simulink model "staubli_20210216_18a"  (R2020a)
settings: Solver=VariableStepAuto  StartTime=0.0  StopTime=10  RelTol=1e-3
values from neighbouring files (symbols this model uses):
  s = T06(1:3,2)    [jacobian_test.m]
undefined symbols (not defined in the file or in its folder): X, Y, Z
libraries: sm_lib x37, nesl_utility x7, dsppolyfun x6, simulink x6
(part 1 of 2)
settings Model: Creator=kdc95  LastModifiedBy=UNIST
settings SolverCC: ZeroCrossAlgorithm=Adaptive
settings DebuggingCC: IgnoredZcDiagnostic=none  ArithmeticOperatorsInVariantConditions=warning
settings SFSimCC: CustomCodeUndefinedFunction=UseInterfaceOnly

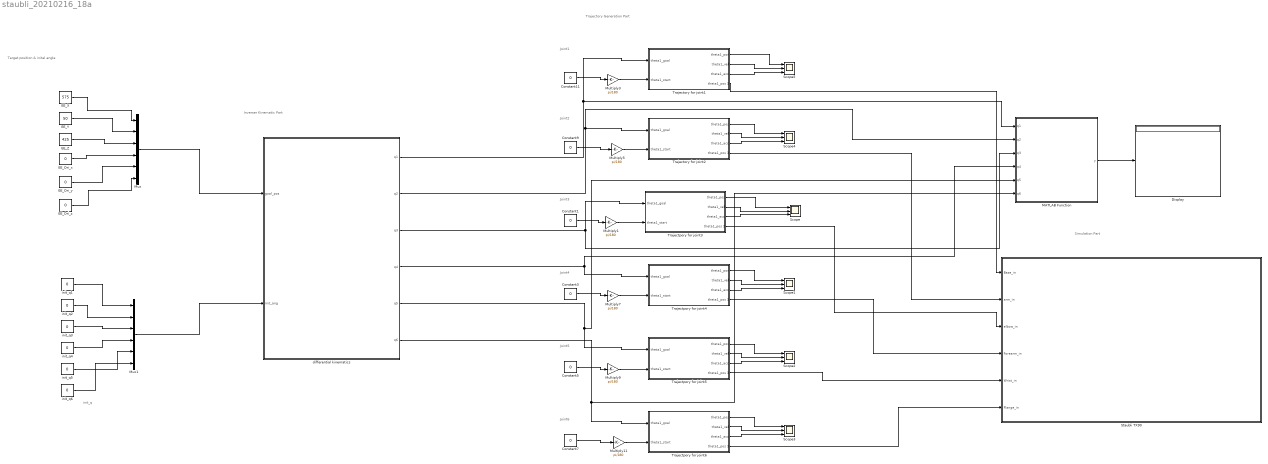
== system staubli_20210216_18a ==
  note: Trajectory Generation Part
  note: init_q
  note: Joint2
  note: Joint3
  note: Joint4
  note: Joint5
  note: Joint1
  note: Joint6
  note: Target position & inital angle
  note: Inverser Kinematic Part
  note: Simulation Part
  Constant{1,3,5,7,9,11} (6 alike) : Constant  Value=0
  Display : Display
  EE_Ori_x : Constant  Value=0
  EE_Ori_y : Constant  Value=0
  EE_Ori_z : Constant  Value=0
  EE_X : Constant  Value=575
  EE_Y : Constant  Value=50
  EE_Z : Constant  Value=425
  MATLAB Function : MATLAB Function  TreatAsAtomicUnit=on
  Multiply{1,3,5,7,9,11} (6 alike) : Gain  Gain=pi/180
  Mux : Mux  Inputs=6
  Mux1 : Mux  Inputs=6
  Scope{,1..5} (6 alike) : Scope  NumInputPorts=3
  Staubli TX90 : Subsystem
      mask Display: image('ROBOT.png'); % Use "Edit Image" on toolstrip to change.
  Trajectory for joint1 : Subsystem
  Trajectory for joint2 : Subsystem
  Trajectpory for joint3 : Subsystem
  Trajectpory for joint4 : Subsystem
  Trajectpory for joint5 : Subsystem
  Trajectpory for joint6 : Subsystem
  differential kinematics : Subsystem
  init_q{1..6} (6 alike) : Constant  Value=0
  wires:
  Trajectpory for joint3/1("theta1_pos ") -> Scope/1
  Trajectory for joint1/3("theta1_acc ") -> Scope5/3
  Trajectpory for joint3/3("theta1_acc ") -> Scope/3
  Constant5/1 -> Multiply9/1
  Trajectpory for joint4/1("theta1_pos ") -> Scope1/1
  Constant11/1 -> Multiply3/1
  Trajectpory for joint5/2("theta1_vel ") -> Scope2/2
  Trajectpory for joint3/2("theta1_vel ") -> Scope/2
  Constant3/1 -> Multiply7/1
  Trajectory for joint1/2("theta1_vel ") -> Scope5/2
  Trajectpory for joint5/1("theta1_pos ") -> Scope2/1
  Trajectpory for joint6/1("theta1_pos ") -> Scope3/1
  Trajectpory for joint5/3("theta1_acc ") -> Scope2/3
  Constant7/1 -> Multiply11/1
  Trajectory for joint2/2("theta1_vel ") -> Scope4/2
  Trajectpory for joint6/3("theta1_acc ") -> Scope3/3
  Trajectory for joint2/1("theta1_pos ") -> Scope4/1
  Trajectory for joint2/3("theta1_acc ") -> Scope4/3
  Trajectpory for joint6/2("theta1_vel ") -> Scope3/2
  Constant1/1 -> Multiply1/1
  Constant9/1 -> Multiply5/1
  Trajectpory for joint4/2("theta1_vel ") -> Scope1/2
  Trajectpory for joint4/3("theta1_acc ") -> Scope1/3
  Trajectory for joint1/1("theta1_pos ") -> Scope5/1
  Trajectory for joint1/4(theta1_pos 1) -> Staubli TX90/1(Base_in)
  Trajectory for joint2/4(theta1_pos 1) -> Staubli TX90/2(arm_in)
  Trajectpory for joint3/4(theta1_pos 1) -> Staubli TX90/3(elbow_in)
  Trajectpory for joint4/4(theta1_pos 1) -> Staubli TX90/4(Forearm_in)
  Trajectpory for joint5/4(theta1_pos 1) -> Staubli TX90/5(Wrist_in)
  Trajectpory for joint6/4(theta1_pos 1) -> Staubli TX90/6(Flange_in)
  differential kinematics/3(q3) -> Trajectpory for joint3/1("theta1_goal "), MATLAB Function/3(q3)
  Multiply1/1 -> Trajectpory for joint3/2("theta1_start ")
  differential kinematics/1(q1) -> Trajectory for joint1/1("theta1_goal "), MATLAB Function/1(q1)
  Multiply3/1 -> Trajectory for joint1/2("theta1_start ")
  differential kinematics/2(q2) -> Trajectory for joint2/1("theta1_goal "), MATLAB Function/2(q2)
  Multiply5/1 -> Trajectory for joint2/2("theta1_start ")
  differential kinematics/4(q4) -> MATLAB Function/4(q4), Trajectpory for joint4/1("theta1_goal ")
  Multiply7/1 -> Trajectpory for joint4/2("theta1_start ")
  differential kinematics/5(q5) -> Trajectpory for joint5/1("theta1_goal "), MATLAB Function/5(q5)
  Multiply9/1 -> Trajectpory for joint5/2("theta1_start ")
  differential kinematics/6(q6) -> Trajectpory for joint6/1("theta1_goal "), MATLAB Function/6(q6)
  Multiply11/1 -> Trajectpory for joint6/2("theta1_start ")
  MATLAB Function/1(y) -> Display/1
  EE_X/1 -> Mux/1
  EE_Y/1 -> Mux/2
  EE_Z/1 -> Mux/3
  EE_Ori_x/1 -> Mux/4
  EE_Ori_y/1 -> Mux/5
  EE_Ori_z/1 -> Mux/6
  init_q1/1 -> Mux1/1
  init_q2/1 -> Mux1/2
  init_q3/1 -> Mux1/3
  init_q4/1 -> Mux1/4
  init_q5/1 -> Mux1/5
  init_q6/1 -> Mux1/6
  Mux/1 -> differential kinematics/1(goal_pos)
  Mux1/1 -> differential kinematics/2(init_ang)

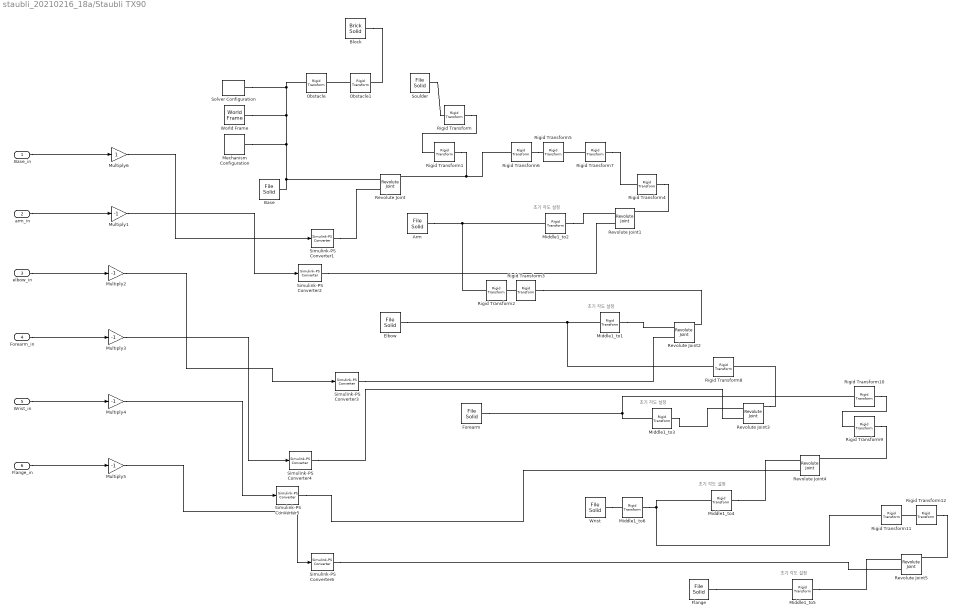
== system staubli_20210216_18a/Staubli TX90 ==
  note: 초기 각도 설정
  note: 초기 각도 설정
  note: 초기 각도 설정
  note: 초기 각도 설정
  note: 초기 각도 설정
  Base_in : Inport
  arm_in : Inport  Port=2
  elbow_in : Inport  Port=3
  Forearm_in : Inport  Port=4
  Wrist_in : Inport  Port=5
  Flange_in : Inport  Port=6
  Arm : sm_lib/Body Elements/File Solid  ExtGeomFileName=C:\Users\UNIST\Desktop\Robot arm\staubli_20210211\arm.stp  UnitType=FromFile  ExtGeomFileUnits=m  StepReaderType=OCC  ExportConvexHullGeometry=off  InertiaType=CalculateFromGeometry  Mass=1  MassUnits=kg  CenterOfMass=[0 0 0]  CenterOfMassUnits=m  MomentsOfInertia=[1 1 1]  MomentsOfInertiaUnits=kg*m^2  ProductsOfInertia=[0 0 0]  ProductsOfInertiaUnits=kg*m^2  BasedOnType=Density  Density=1000  DensityUnits=kg/m^3  DoExposeReferenceFrame=on  SerializedFrames=<Frames/>  GraphicType=FromGeometry  MarkerShape=Sphere  MarkerSize=10  GraphicVisPropType=SimpleVisualProperties  GraphicDiffuseColor=[1.0 1.0 1.0]  GraphicSpecularColor=[0.5 0.5 0.5 1.0]  GraphicAmbientColor=[0.15 0.15 0.15 1.0]  GraphicEmissiveColor=[0.0 0.0 0.0 1.0]  GraphicShininess=75  GraphicOpacity=1
  Base : sm_lib/Body Elements/File Solid  ExtGeomFileName=C:\Users\UNIST\Desktop\Robot arm\staubli_20210211\Base.stp  UnitType=FromFile  ExtGeomFileUnits=m  StepReaderType=HEX  ExportConvexHullGeometry=off  InertiaType=CalculateFromGeometry  Mass=1  MassUnits=kg  CenterOfMass=[0 0 0]  CenterOfMassUnits=m  MomentsOfInertia=[1 1 1]  MomentsOfInertiaUnits=kg*m^2  ProductsOfInertia=[0 0 0]  ProductsOfInertiaUnits=kg*m^2  BasedOnType=Density  Density=1000  DensityUnits=kg/m^3  DoExposeReferenceFrame=on  SerializedFrames=<Frames/>  GraphicType=FromGeometry  MarkerShape=Sphere  MarkerSize=10  GraphicVisPropType=SimpleVisualProperties  GraphicDiffuseColor=[0.5 0.5 0.5]  GraphicSpecularColor=[0.5 0.5 0.5 1.0]  GraphicAmbientColor=[0.15 0.15 0.15 1.0]  GraphicEmissiveColor=[0.0 0.0 0.0 1.0]  GraphicShininess=75  GraphicOpacity=1.0
  Block : sm_lib/Body Elements/Brick Solid  GraphicAmbientColor=[0.15 0.15 0.15 1.0]  BasedOnType=Density  BrickDimensions=[550 400 100]  BrickDimensionUnits=mm  CenterOfMass=[0 0 0]  CenterOfMassUnits=m  GraphicDiffuseColor=[0.5 0.5 0.5]  Density=1000  DensityUnits=kg/m^3  DoExposeReferenceFrame=on  GraphicEmissiveColor=[0.0 0.0 0.0 1.0]  ExportEntireGeometry=off  SerializedFrames=<Frames/>  MarkerShape=Sphere  MarkerSize=10  GraphicType=FromGeometry  InertiaType=CalculateFromGeometry  Mass=1  MassUnits=kg  MomentsOfInertia=[1 1 1]  MomentsOfInertiaUnits=kg*m^2  GraphicOpacity=1.0  ProductsOfInertia=[0 0 0]  ProductsOfInertiaUnits=kg*m^2  GraphicShininess=75  GraphicSpecularColor=[0.5 0.5 0.5 1.0]  GraphicVisPropType=SimpleVisualProperties
  Elbow : sm_lib/Body Elements/File Solid  ExtGeomFileName=C:\Users\UNIST\Desktop\Robot arm\staubli_20210211\Elbow.stp  UnitType=FromFile  ExtGeomFileUnits=m  StepReaderType=OCC  ExportConvexHullGeometry=off  InertiaType=CalculateFromGeometry  Mass=1  MassUnits=kg  CenterOfMass=[0 0 0]  CenterOfMassUnits=m  MomentsOfInertia=[1 1 1]  MomentsOfInertiaUnits=kg*m^2  ProductsOfInertia=[0 0 0]  ProductsOfInertiaUnits=kg*m^2  BasedOnType=Density  Density=1000  DensityUnits=kg/m^3  DoExposeReferenceFrame=on  SerializedFrames=<Frames/>  GraphicType=FromGeometry  MarkerShape=Sphere  MarkerSize=10  GraphicVisPropType=SimpleVisualProperties  GraphicDiffuseColor=[1.0 1.0 1.0]  GraphicSpecularColor=[0.5 0.5 0.5 1.0]  GraphicAmbientColor=[0.15 0.15 0.15 1.0]  GraphicEmissiveColor=[0.0 0.0 0.0 1.0]  GraphicShininess=75  GraphicOpacity=1
  Flange : sm_lib/Body Elements/File Solid  ExtGeomFileName=C:\Users\UNIST\Desktop\Robot arm\staubli_20210211\Flange.stp  UnitType=FromFile  ExtGeomFileUnits=m  StepReaderType=OCC  ExportConvexHullGeometry=off  InertiaType=CalculateFromGeometry  Mass=1  MassUnits=kg  CenterOfMass=[0 0 0]  CenterOfMassUnits=m  MomentsOfInertia=[1 1 1]  MomentsOfInertiaUnits=kg*m^2  ProductsOfInertia=[0 0 0]  ProductsOfInertiaUnits=kg*m^2  BasedOnType=Density  Density=1000  DensityUnits=kg/m^3  DoExposeReferenceFrame=on  SerializedFrames=<Frames/>  GraphicType=FromGeometry  MarkerShape=Sphere  MarkerSize=10  GraphicVisPropType=SimpleVisualProperties  GraphicDiffuseColor=[1.0 1.0 1.0]  GraphicSpecularColor=[0.5 0.5 0.5 1.0]  GraphicAmbientColor=[0.15 0.15 0.15 1.0]  GraphicEmissiveColor=[0.0 0.0 0.0 1.0]  GraphicShininess=75  GraphicOpacity=1
  Forearm : sm_lib/Body Elements/File Solid  ExtGeomFileName=C:\Users\UNIST\Desktop\Robot arm\staubli_20210211\Forearm.stp  UnitType=FromFile  ExtGeomFileUnits=m  StepReaderType=OCC  ExportConvexHullGeometry=off  InertiaType=CalculateFromGeometry  Mass=1  MassUnits=kg  CenterOfMass=[0 0 0]  CenterOfMassUnits=m  MomentsOfInertia=[1 1 1]  MomentsOfInertiaUnits=kg*m^2  ProductsOfInertia=[0 0 0]  ProductsOfInertiaUnits=kg*m^2  BasedOnType=Density  Density=1000  DensityUnits=kg/m^3  DoExposeReferenceFrame=on  SerializedFrames=<Frames/>  GraphicType=FromGeometry  MarkerShape=Sphere  MarkerSize=10  GraphicVisPropType=SimpleVisualProperties  GraphicDiffuseColor=[1.0 1.0 1.0]  GraphicSpecularColor=[0.5 0.5 0.5 1.0]  GraphicAmbientColor=[0.15 0.15 0.15 1.0]  GraphicEmissiveColor=[0.0 0.0 0.0 1.0]  GraphicShininess=75  GraphicOpacity=1
  Mechanism Configuration : sm_lib/Utilities/Mechanism Configuration  UniformGravity=Constant  GravityVector=[0 0 -9.80665]  GravityUnits=m/s^2  LinearizationDelta=0.001
  Middle1_to1 : sm_lib/Frames and Transforms/Rigid Transform  TranslationMethod=None  TranslationStandardOffset=45  TranslationLengthUnit=mm  TranslationStandardAxis=+Z  TranslationCartesianOffset=[0 0 0]  TranslationROffset=0  TranslationROffsetUnits=m  TranslationZOffset=0  TranslationZOffsetUnits=m  TranslationThetaOffset=0  TranslationThetaOffsetUnits=deg  RotationMethod=StandardAxis  RotationAngleUnits=deg  RotationStandardAxis=-Z  RotationAngle=0  RotationArbitraryAxis=[0 0 1]  FollAlignAxisA=+X  BaseAlignAxisA=+Y  FollAlignAxisB=+Y  BaseAlignAxisB=+Z  RotationSequenceAxes=FollowerAxes  RotationSequence=XYX  RotationSequenceAngles=[0 0 0]  RotationSequenceAnglesUnits=deg  RotationMatrix=[1 0 0; 0 1 0; 0 0 1]
  Middle1_to2 : sm_lib/Frames and Transforms/Rigid Transform  TranslationMethod=None  TranslationStandardOffset=45  TranslationLengthUnit=mm  TranslationStandardAxis=+Z  TranslationCartesianOffset=[0 0 0]  TranslationROffset=0  TranslationROffsetUnits=m  TranslationZOffset=0  TranslationZOffsetUnits=m  TranslationThetaOffset=0  TranslationThetaOffsetUnits=deg  RotationMethod=None  RotationAngleUnits=deg  RotationStandardAxis=+Z  RotationAngle=0  RotationArbitraryAxis=[0 0 1]  FollAlignAxisA=+X  BaseAlignAxisA=+Y  FollAlignAxisB=+Y  BaseAlignAxisB=+Z  RotationSequenceAxes=FollowerAxes  RotationSequence=XYX  RotationSequenceAngles=[0 0 0]  RotationSequenceAnglesUnits=deg  RotationMatrix=[1 0 0; 0 1 0; 0 0 1]
  Middle1_to3 : sm_lib/Frames and Transforms/Rigid Transform  TranslationMethod=None  TranslationStandardOffset=45  TranslationLengthUnit=mm  TranslationStandardAxis=+Z  TranslationCartesianOffset=[0 0 0]  TranslationROffset=0  TranslationROffsetUnits=m  TranslationZOffset=0  TranslationZOffsetUnits=m  TranslationThetaOffset=0  TranslationThetaOffsetUnits=deg  RotationMethod=None  RotationAngleUnits=deg  RotationStandardAxis=+Z  RotationAngle=-90  RotationArbitraryAxis=[0 0 1]  FollAlignAxisA=+X  BaseAlignAxisA=+Y  FollAlignAxisB=+Y  BaseAlignAxisB=+Z  RotationSequenceAxes=FollowerAxes  RotationSequence=XYX  RotationSequenceAngles=[0 0 0]  RotationSequenceAnglesUnits=deg  RotationMatrix=[1 0 0; 0 1 0; 0 0 1]
  Middle1_to4 : sm_lib/Frames and Transforms/Rigid Transform  TranslationMethod=None  TranslationStandardOffset=45  TranslationLengthUnit=mm  TranslationStandardAxis=+Z  TranslationCartesianOffset=[0 0 0]  TranslationROffset=0  TranslationROffsetUnits=m  TranslationZOffset=0  TranslationZOffsetUnits=m  TranslationThetaOffset=0  TranslationThetaOffsetUnits=deg  RotationMethod=None  RotationAngleUnits=deg  RotationStandardAxis=-Z  RotationAngle=-90  RotationArbitraryAxis=[0 0 1]  FollAlignAxisA=+X  BaseAlignAxisA=+Y  FollAlignAxisB=+Y  BaseAlignAxisB=+Z  RotationSequenceAxes=FollowerAxes  RotationSequence=XYX  RotationSequenceAngles=[0 0 0]  RotationSequenceAnglesUnits=deg  RotationMatrix=[1 0 0; 0 1 0; 0 0 1]
  Middle1_to5 : sm_lib/Frames and Transforms/Rigid Transform  TranslationMethod=None  TranslationStandardOffset=45  TranslationLengthUnit=mm  TranslationStandardAxis=+Z  TranslationCartesianOffset=[0 0 0]  TranslationROffset=0  TranslationROffsetUnits=m  TranslationZOffset=0  TranslationZOffsetUnits=m  TranslationThetaOffset=0  TranslationThetaOffsetUnits=deg  RotationMethod=None  RotationAngleUnits=deg  RotationStandardAxis=+Z  RotationAngle=-90  RotationArbitraryAxis=[0 0 1]  FollAlignAxisA=+X  BaseAlignAxisA=+Y  FollAlignAxisB=+Y  BaseAlignAxisB=+Z  RotationSequenceAxes=FollowerAxes  RotationSequence=XYX  RotationSequenceAngles=[0 0 0]  RotationSequenceAnglesUnits=deg  RotationMatrix=[1 0 0; 0 1 0; 0 0 1]
  Middle1_to6 : sm_lib/Frames and Transforms/Rigid Transform  TranslationMethod=None  TranslationStandardOffset=45  TranslationLengthUnit=mm  TranslationStandardAxis=+Z  TranslationCartesianOffset=[0 0 0]  TranslationROffset=0  TranslationROffsetUnits=m  TranslationZOffset=0  TranslationZOffsetUnits=m  TranslationThetaOffset=0  TranslationThetaOffsetUnits=deg  RotationMethod=StandardAxis  RotationAngleUnits=deg  RotationStandardAxis=+Z  RotationAngle=-90  RotationArbitraryAxis=[0 0 1]  FollAlignAxisA=+X  BaseAlignAxisA=+Y  FollAlignAxisB=+Y  BaseAlignAxisB=+Z  RotationSequenceAxes=FollowerAxes  RotationSequence=XYX  RotationSequenceAngles=[0 0 0]  RotationSequenceAnglesUnits=deg  RotationMatrix=[1 0 0; 0 1 0; 0 0 1]
  Multiply{1..5} (5 alike) : Gain  Gain=-1
  Multiply6 : Gain
  Obstacle : sm_lib/Frames and Transforms/Rigid Transform  TranslationMethod=StandardAxis  TranslationStandardOffset=700  TranslationLengthUnit=mm  TranslationStandardAxis=+X  TranslationCartesianOffset=[0 0 0]  TranslationROffset=0  TranslationROffsetUnits=m  TranslationZOffset=0  TranslationZOffsetUnits=m  TranslationThetaOffset=0  TranslationThetaOffsetUnits=deg  RotationMethod=None  RotationAngleUnits=deg  RotationStandardAxis=-X  RotationAngle=90  RotationArbitraryAxis=[0 0 1]  FollAlignAxisA=+X  BaseAlignAxisA=+Y  FollAlignAxisB=+Y  BaseAlignAxisB=+Z  RotationSequenceAxes=FollowerAxes  RotationSequence=XYX  RotationSequenceAngles=[0 0 0]  RotationSequenceAnglesUnits=deg  RotationMatrix=[1 0 0; 0 1 0; 0 0 1]
  Obstacle1 : sm_lib/Frames and Transforms/Rigid Transform  TranslationMethod=StandardAxis  TranslationStandardOffset=50  TranslationLengthUnit=mm  TranslationStandardAxis=+Z  TranslationCartesianOffset=[0 0 0]  TranslationROffset=0  TranslationROffsetUnits=m  TranslationZOffset=0  TranslationZOffsetUnits=m  TranslationThetaOffset=0  TranslationThetaOffsetUnits=deg  RotationMethod=None  RotationAngleUnits=deg  RotationStandardAxis=-X  RotationAngle=90  RotationArbitraryAxis=[0 0 1]  FollAlignAxisA=+X  BaseAlignAxisA=+Y  FollAlignAxisB=+Y  BaseAlignAxisB=+Z  RotationSequenceAxes=FollowerAxes  RotationSequence=XYX  RotationSequenceAngles=[0 0 0]  RotationSequenceAnglesUnits=deg  RotationMatrix=[1 0 0; 0 1 0; 0 0 1]
  Revolute Joint{,1..5} (6 alike) : sm_lib/Joints/Revolute Joint  JointMode=Normal  SenseConstraintForce=off  SenseConstraintForceX=off  SenseConstraintForceY=off  SenseConstraintForceZ=off  SenseConstraintTorque=off  SenseConstraintTorqueX=off  SenseConstraintTorqueY=off  SenseConstraintTorqueZ=off  SenseTotalForce=off  SenseTotalForceX=off  SenseTotalForceY=off  SenseTotalForceZ=off  SenseTotalTorque=off  SenseTotalTorqueX=off  SenseTotalTorqueY=off  SenseTotalTorqueZ=off  CompositeWrenchDir=FollowerOnBase  CompositeWrenchFrame=BaseFrame  EquilibriumPosition=0  EquilibriumPositionUnits=deg  SpringStiffness=0  SpringStiffnessUnits=N*m/deg  DampingCoefficient=0.1  DampingCoefficientUnits=N*m/(deg/s)  TorqueActuationMode=ComputedTorque  MotionActuationMode=InputMotion  SensePosition=on  SenseVelocity=off  SenseAcceleration=off  SenseTorqueForce=on  SenseLowerLimitTorqueForce=off  SenseUpperLimitTorqueForce=off  LowerLimitSpecify=off  LowerLimitBound=-90  LowerLimitBoundUnits=deg  LowerLimitStiffness=1e4  LowerLimitStiffnessUnits=N*m/deg  LowerLimitDamping=10  LowerLimitDampingUnits=N*m/(deg/s)  LowerLimitTransitionRegionWidth=0.1  LowerLimitTransitionRegionWidthUnits=deg  UpperLimitSpecify=off  UpperLimitBound=90  UpperLimitBoundUnits=deg  UpperLimitStiffness=1e4  UpperLimitStiffnessUnits=N*m/deg  UpperLimitDamping=10  UpperLimitDampingUnits=N*m/(deg/s)  UpperLimitTransitionRegionWidth=0.1  UpperLimitTransitionRegionWidthUnits=deg  PositionTargetSpecify=off  PositionTargetPriority=High  PositionTargetValue=0  PositionTargetValueUnits=deg  VelocityTargetSpecify=off  VelocityTargetPriority=High  VelocityTargetValue=0  VelocityTargetValueUnits=deg/s
  Rigid Transform : sm_lib/Frames and Transforms/Rigid Transform  TranslationMethod=StandardAxis  TranslationStandardOffset=478  TranslationLengthUnit=mm  TranslationStandardAxis=-Z  TranslationCartesianOffset=[0 0 0]  TranslationROffset=0  TranslationROffsetUnits=m  TranslationZOffset=0  TranslationZOffsetUnits=m  TranslationThetaOffset=0  TranslationThetaOffsetUnits=deg  RotationMethod=None  RotationAngleUnits=deg  RotationStandardAxis=+Z  RotationAngle=0.0  RotationArbitraryAxis=[0 0 1]  FollAlignAxisA=+X  BaseAlignAxisA=+Y  FollAlignAxisB=+Y  BaseAlignAxisB=+Z  RotationSequenceAxes=FollowerAxes  RotationSequence=XYX  RotationSequenceAngles=[0 0 0]  RotationSequenceAnglesUnits=deg  RotationMatrix=[1 0 0; 0 1 0; 0 0 1]
  Rigid Transform1 : sm_lib/Frames and Transforms/Rigid Transform  TranslationMethod=None  TranslationStandardOffset=50  TranslationLengthUnit=mm  TranslationStandardAxis=-X  TranslationCartesianOffset=[0 0 0]  TranslationROffset=0  TranslationROffsetUnits=m  TranslationZOffset=0  TranslationZOffsetUnits=m  TranslationThetaOffset=0  TranslationThetaOffsetUnits=deg  RotationMethod=None  RotationAngleUnits=deg  RotationStandardAxis=+Z  RotationAngle=0.0  RotationArbitraryAxis=[0 0 1]  FollAlignAxisA=+X  BaseAlignAxisA=+Y  FollAlignAxisB=+Y  BaseAlignAxisB=+Z  RotationSequenceAxes=FollowerAxes  RotationSequence=XYX  RotationSequenceAngles=[0 0 0]  RotationSequenceAnglesUnits=deg  RotationMatrix=[1 0 0; 0 1 0; 0 0 1]
  Rigid Transform10 : sm_lib/Frames and Transforms/Rigid Transform  TranslationMethod=None  TranslationStandardOffset=425  TranslationLengthUnit=mm  TranslationStandardAxis=-Y  TranslationCartesianOffset=[0 0 0]  TranslationROffset=0  TranslationROffsetUnits=m  TranslationZOffset=0  TranslationZOffsetUnits=m  TranslationThetaOffset=0  TranslationThetaOffsetUnits=deg  RotationMethod=StandardAxis  RotationAngleUnits=deg  RotationStandardAxis=-X  RotationAngle=90  RotationArbitraryAxis=[0 0 1]  FollAlignAxisA=+X  BaseAlignAxisA=+Y  FollAlignAxisB=+Y  BaseAlignAxisB=+Z  RotationSequenceAxes=FollowerAxes  RotationSequence=XYX  RotationSequenceAngles=[0 0 0]  RotationSequenceAnglesUnits=deg  RotationMatrix=[1 0 0; 0 1 0; 0 0 1]
  Rigid Transform11 : sm_lib/Frames and Transforms/Rigid Transform  TranslationMethod=None  TranslationStandardOffset=425  TranslationLengthUnit=mm  TranslationStandardAxis=-Y  TranslationCartesianOffset=[0 0 0]  TranslationROffset=0  TranslationROffsetUnits=m  TranslationZOffset=0  TranslationZOffsetUnits=m  TranslationThetaOffset=0  TranslationThetaOffsetUnits=deg  RotationMethod=StandardAxis  RotationAngleUnits=deg  RotationStandardAxis=+X  RotationAngle=90  RotationArbitraryAxis=[0 0 1]  FollAlignAxisA=+X  BaseAlignAxisA=+Y  FollAlignAxisB=+Y  BaseAlignAxisB=+Z  RotationSequenceAxes=FollowerAxes  RotationSequence=XYX  RotationSequenceAngles=[0 0 0]  RotationSequenceAnglesUnits=deg  RotationMatrix=[1 0 0; 0 1 0; 0 0 1]
  Rigid Transform12 : sm_lib/Frames and Transforms/Rigid Transform  TranslationMethod=StandardAxis  TranslationStandardOffset=100  TranslationLengthUnit=mm  TranslationStandardAxis=+Z  TranslationCartesianOffset=[0 0 0]  TranslationROffset=0  TranslationROffsetUnits=m  TranslationZOffset=0  TranslationZOffsetUnits=m  TranslationThetaOffset=0  TranslationThetaOffsetUnits=deg  RotationMethod=None  RotationAngleUnits=deg  RotationStandardAxis=+Z  RotationAngle=425  RotationArbitraryAxis=[0 0 1]  FollAlignAxisA=+X  BaseAlignAxisA=+Y  FollAlignAxisB=+Y  BaseAlignAxisB=+Z  RotationSequenceAxes=FollowerAxes  RotationSequence=XYX  RotationSequenceAngles=[0 0 0]  RotationSequenceAnglesUnits=deg  RotationMatrix=[1 0 0; 0 1 0; 0 0 1]
  Rigid Transform2 : sm_lib/Frames and Transforms/Rigid Transform  TranslationMethod=StandardAxis  TranslationStandardOffset=425  TranslationLengthUnit=mm  TranslationStandardAxis=-Y  TranslationCartesianOffset=[0 0 0]  TranslationROffset=0  TranslationROffsetUnits=m  TranslationZOffset=0  TranslationZOffsetUnits=m  TranslationThetaOffset=0  TranslationThetaOffsetUnits=deg  RotationMethod=None  RotationAngleUnits=deg  RotationStandardAxis=+X  RotationAngle=90  RotationArbitraryAxis=[0 0 1]  FollAlignAxisA=+X  BaseAlignAxisA=+Y  FollAlignAxisB=+Y  BaseAlignAxisB=+Z  RotationSequenceAxes=FollowerAxes  RotationSequence=XYX  RotationSequenceAngles=[0 0 0]  RotationSequenceAnglesUnits=deg  RotationMatrix=[1 0 0; 0 1 0; 0 0 1]
  Rigid Transform3 : sm_lib/Frames and Transforms/Rigid Transform  TranslationMethod=StandardAxis  TranslationStandardOffset=50  TranslationLengthUnit=mm  TranslationStandardAxis=+Z  TranslationCartesianOffset=[0 0 0]  TranslationROffset=0  TranslationROffsetUnits=m  TranslationZOffset=0  TranslationZOffsetUnits=m  TranslationThetaOffset=0  TranslationThetaOffsetUnits=deg  RotationMethod=None  RotationAngleUnits=deg  RotationStandardAxis=+X  RotationAngle=90  RotationArbitraryAxis=[0 0 1]  FollAlignAxisA=+X  BaseAlignAxisA=+Y  FollAlignAxisB=+Y  BaseAlignAxisB=+Z  RotationSequenceAxes=FollowerAxes  RotationSequence=XYX  RotationSequenceAngles=[0 0 0]  RotationSequenceAnglesUnits=deg  RotationMatrix=[1 0 0; 0 1 0; 0 0 1]
  Rigid Transform4 : sm_lib/Frames and Transforms/Rigid Transform  TranslationMethod=StandardAxis  TranslationStandardOffset=50  TranslationLengthUnit=mm  TranslationStandardAxis=+X  TranslationCartesianOffset=[0 0 0]  TranslationROffset=0  TranslationROffsetUnits=m  TranslationZOffset=0  TranslationZOffsetUnits=m  TranslationThetaOffset=0  TranslationThetaOffsetUnits=deg  RotationMethod=None  RotationAngleUnits=deg  RotationStandardAxis=+X  RotationAngle=90  RotationArbitraryAxis=[0 0 1]  FollAlignAxisA=+X  BaseAlignAxisA=+Y  FollAlignAxisB=+Y  BaseAlignAxisB=+Z  RotationSequenceAxes=FollowerAxes  RotationSequence=XYX  RotationSequenceAngles=[0 0 0]  RotationSequenceAnglesUnits=deg  RotationMatrix=[1 0 0; 0 1 0; 0 0 1]
  Rigid Transform5 : sm_lib/Frames and Transforms/Rigid Transform  TranslationMethod=StandardAxis  TranslationStandardOffset=425  TranslationLengthUnit=mm  TranslationStandardAxis=-Y  TranslationCartesianOffset=[0 0 0]  TranslationROffset=0  TranslationROffsetUnits=m  TranslationZOffset=0  TranslationZOffsetUnits=m  TranslationThetaOffset=0  TranslationThetaOffsetUnits=deg  RotationMethod=None  RotationAngleUnits=deg  RotationStandardAxis=+X  RotationAngle=90  RotationArbitraryAxis=[0 0 1]  FollAlignAxisA=+X  BaseAlignAxisA=+Y  FollAlignAxisB=+Y  BaseAlignAxisB=+Z  RotationSequenceAxes=FollowerAxes  RotationSequence=XYX  RotationSequenceAngles=[0 0 0]  RotationSequenceAnglesUnits=deg  RotationMatrix=[1 0 0; 0 1 0; 0 0 1]
  Rigid Transform6 : sm_lib/Frames and Transforms/Rigid Transform  TranslationMethod=None  TranslationStandardOffset=50  TranslationLengthUnit=mm  TranslationStandardAxis=-X  TranslationCartesianOffset=[0 0 0]  TranslationROffset=0  TranslationROffsetUnits=m  TranslationZOffset=0  TranslationZOffsetUnits=m  TranslationThetaOffset=0  TranslationThetaOffsetUnits=deg  RotationMethod=StandardAxis  RotationAngleUnits=deg  RotationStandardAxis=-X  RotationAngle=90  RotationArbitraryAxis=[0 0 1]  FollAlignAxisA=+X  BaseAlignAxisA=+Y  FollAlignAxisB=+Y  BaseAlignAxisB=+Z  RotationSequenceAxes=FollowerAxes  RotationSequence=XYX  RotationSequenceAngles=[0 0 0]  RotationSequenceAnglesUnits=deg  RotationMatrix=[1 0 0; 0 1 0; 0 0 1]
  Rigid Transform7 : sm_lib/Frames and Transforms/Rigid Transform  TranslationMethod=StandardAxis  TranslationStandardOffset=50  TranslationLengthUnit=mm  TranslationStandardAxis=-Y  TranslationCartesianOffset=[0 0 0]  TranslationROffset=0  TranslationROffsetUnits=m  TranslationZOffset=0  TranslationZOffsetUnits=m  TranslationThetaOffset=0  TranslationThetaOffsetUnits=deg  RotationMethod=None  RotationAngleUnits=deg  RotationStandardAxis=+X  RotationAngle=90  RotationArbitraryAxis=[0 0 1]  FollAlignAxisA=+X  BaseAlignAxisA=+Y  FollAlignAxisB=+Y  BaseAlignAxisB=+Z  RotationSequenceAxes=FollowerAxes  RotationSequence=XYX  RotationSequenceAngles=[0 0 0]  RotationSequenceAnglesUnits=deg  RotationMatrix=[1 0 0; 0 1 0; 0 0 1]
  Rigid Transform8 : sm_lib/Frames and Transforms/Rigid Transform  TranslationMethod=None  TranslationStandardOffset=425  TranslationLengthUnit=mm  TranslationStandardAxis=-Y  TranslationCartesianOffset=[0 0 0]  TranslationROffset=0  TranslationROffsetUnits=m  TranslationZOffset=0  TranslationZOffsetUnits=m  TranslationThetaOffset=0  TranslationThetaOffsetUnits=deg  RotationMethod=StandardAxis  RotationAngleUnits=deg  RotationStandardAxis=+X  RotationAngle=90  RotationArbitraryAxis=[0 0 1]  FollAlignAxisA=+X  BaseAlignAxisA=+Y  FollAlignAxisB=+Y  BaseAlignAxisB=+Z  RotationSequenceAxes=FollowerAxes  RotationSequence=XYX  RotationSequenceAngles=[0 0 0]  RotationSequenceAnglesUnits=deg  RotationMatrix=[1 0 0; 0 1 0; 0 0 1]
  Rigid Transform9 : sm_lib/Frames and Transforms/Rigid Transform  TranslationMethod=StandardAxis  TranslationStandardOffset=425  TranslationLengthUnit=mm  TranslationStandardAxis=-Y  TranslationCartesianOffset=[0 0 0]  TranslationROffset=0  TranslationROffsetUnits=m  TranslationZOffset=0  TranslationZOffsetUnits=m  TranslationThetaOffset=0  TranslationThetaOffsetUnits=deg  RotationMethod=None  RotationAngleUnits=deg  RotationStandardAxis=+Z  RotationAngle=425  RotationArbitraryAxis=[0 0 1]  FollAlignAxisA=+X  BaseAlignAxisA=+Y  FollAlignAxisB=+Y  BaseAlignAxisB=+Z  RotationSequenceAxes=FollowerAxes  RotationSequence=XYX  RotationSequenceAngles=[0 0 0]  RotationSequenceAnglesUnits=deg  RotationMatrix=[1 0 0; 0 1 0; 0 0 1]
  Simulink-PS Converter{1..6} (6 alike) : nesl_utility/Simulink-PS Converter  PhysicalDomain=network_engine_domain  SubClassName=ps_input  LeftPortType=input  RightPortType=output  PseudoPeriodic=off  Frequencies=[]  NoiseDistribution=none  NoiseParameters=[]  Unit=1  AffineConversion=off  FilteringAndDerivatives=filter  SimscapeFilterOrder=2  InputFilterTimeConstant=0.1  UdotUserProvided=0
  Solver Configuration : nesl_utility/Solver Configuration  PhysicalDomain=network_engine_domain  SubClassName=solver  LeftPortType=input  RightPortType=generic  Tones=[]  Harmonics=[]  SimulateNoise=off  Profile=off  UseLocalSampling=off  EnableSwitchedLinearOptims=on  FrequencyDomain=off  UseCCode=off  RelTol=0.001  AbsTol=1e-06  MinStep=1e-09  ToWorkspace=off  RevertToSquareIcSolve=off  NumHomotopyIterations=100  PhasorMode=off  PhasorModeNumHarmonics=1  DoDC=off  ResidualTolerance=1e-09  UseLocalSolver=off  LocalSolverChoice=NE_BACKWARD_EULER_ADVANCER  LocalSolverSampleTime=0.001  DoFixedCost=off  MaxNonlinIter=3  MaxModeIter=2  LinearAlgebra=auto  EquationFormulation=NE_TIME_EF  DelaysMemoryBudget=1024  AutomaticFiltering=on  FilteringTimeConstant=0.001  PartitionStorageMethod=AS_NEEDED  PartitionMemoryBudget=1024  PartitionMethod=ROBUST
  Soulder : sm_lib/Body Elements/File Solid  ExtGeomFileName=C:\Users\UNIST\Desktop\Robot arm\staubli_20210211\Shoulder.stp  UnitType=FromFile  ExtGeomFileUnits=m  StepReaderType=HEX  ExportConvexHullGeometry=off  InertiaType=CalculateFromGeometry  Mass=1  MassUnits=kg  CenterOfMass=[0 0 0]  CenterOfMassUnits=m  MomentsOfInertia=[1 1 1]  MomentsOfInertiaUnits=kg*m^2  ProductsOfInertia=[0 0 0]  ProductsOfInertiaUnits=kg*m^2  BasedOnType=Density  Density=1000  DensityUnits=kg/m^3  DoExposeReferenceFrame=on  SerializedFrames=<Frames/>  GraphicType=FromGeometry  MarkerShape=Sphere  MarkerSize=10  GraphicVisPropType=SimpleVisualProperties  GraphicDiffuseColor=[0.5 0.5 0.5]  GraphicSpecularColor=[0.5 0.5 0.5 1.0]  GraphicAmbientColor=[0.15 0.15 0.15 1.0]  GraphicEmissiveColor=[0.0 0.0 0.0 1.0]  GraphicShininess=75  GraphicOpacity=1.0
  World Frame : sm_lib/Frames and Transforms/World Frame
  Wrist : sm_lib/Body Elements/File Solid  ExtGeomFileName=C:\Users\UNIST\Desktop\Robot arm\staubli_20210211\Wrist.stp  UnitType=FromFile  ExtGeomFileUnits=m  StepReaderType=OCC  ExportConvexHullGeometry=off  InertiaType=CalculateFromGeometry  Mass=1  MassUnits=kg  CenterOfMass=[0 0 0]  CenterOfMassUnits=m  MomentsOfInertia=[1 1 1]  MomentsOfInertiaUnits=kg*m^2  ProductsOfInertia=[0 0 0]  ProductsOfInertiaUnits=kg*m^2  BasedOnType=Density  Density=1000  DensityUnits=kg/m^3  DoExposeReferenceFrame=on  SerializedFrames=<Frames/>  GraphicType=FromGeometry  MarkerShape=Sphere  MarkerSize=10  GraphicVisPropType=SimpleVisualProperties  GraphicDiffuseColor=[1.0 1.0 1.0]  GraphicSpecularColor=[0.5 0.5 0.5 1.0]  GraphicAmbientColor=[0.15 0.15 0.15 1.0]  GraphicEmissiveColor=[0.0 0.0 0.0 1.0]  GraphicShininess=75  GraphicOpacity=1
  wires:
  arm_in/1 -> Multiply1/1
  elbow_in/1 -> Multiply2/1
  Wrist_in/1 -> Multiply4/1
  Forearm_in/1 -> Multiply3/1
  Base_in/1 -> Multiply6/1
  Multiply1/1 -> Simulink-PS Converter2/1
  Multiply2/1 -> Simulink-PS Converter3/1
  Multiply3/1 -> Simulink-PS Converter4/1
  Multiply4/1 -> Simulink-PS Converter5/1
  Multiply5/1 -> Simulink-PS Converter6/1
  Flange_in/1 -> Multiply5/1
  Multiply6/1 -> Simulink-PS Converter1/1
  connections:
  Solver Configuration/RConn1 -- Revolute Joint/LConn1 -- Base/RConn1 -- Mechanism Configuration/RConn1 -- World Frame/RConn1 -- Obstacle/LConn1
  Block/RConn1 -- Obstacle1/RConn1
  Obstacle1/LConn1 -- Obstacle/RConn1
  Simulink-PS Converter1/RConn1 -- Revolute Joint/LConn2
  Soulder/RConn1 -- Rigid Transform/LConn1
  Rigid Transform/RConn1 -- Rigid Transform1/LConn1
  Rigid Transform1/RConn1 -- Revolute Joint/RConn1 -- Rigid Transform6/LConn1
  Arm/RConn1 -- Rigid Transform2/LConn1 -- Middle1_to2/LConn1
  Simulink-PS Converter2/RConn1 -- Revolute Joint1/LConn2
  Middle1_to2/RConn1 -- Revolute Joint1/LConn1
  Rigid Transform7/LConn1 -- Rigid Transform5/RConn1
  Rigid Transform6/RConn1 -- Rigid Transform5/LConn1
  Rigid Transform7/RConn1 -- Rigid Transform4/LConn1
  Rigid Transform4/RConn1 -- Revolute Joint1/RConn1
  Elbow/RConn1 -- Rigid Transform8/LConn1 -- Middle1_to1/LConn1
  Rigid Transform3/LConn1 -- Rigid Transform2/RConn1
  Rigid Transform3/RConn1 -- Revolute Joint2/RConn1
  Simulink-PS Converter3/RConn1 -- Revolute Joint2/LConn2
  Middle1_to1/RConn1 -- Revolute Joint2/LConn1
  Forearm/RConn1 -- Middle1_to3/LConn1 -- Rigid Transform10/LConn1
  Middle1_to3/RConn1 -- Revolute Joint3/LConn1
  Revolute Joint3/RConn1 -- Rigid Transform8/RConn1
  Rigid Transform11/LConn1 -- Middle1_to6/RConn1 -- Middle1_to4/LConn1
  Rigid Transform10/RConn1 -- Rigid Transform9/LConn1
  Rigid Transform9/RConn1 -- Revolute Joint4/RConn1
  Middle1_to5/RConn1 -- Revolute Joint5/LConn1
  Flange/RConn1 -- Middle1_to5/LConn1
  Rigid Transform12/LConn1 -- Rigid Transform11/RConn1
  Rigid Transform12/RConn1 -- Revolute Joint5/RConn1
  Simulink-PS Converter4/RConn1 -- Revolute Joint3/LConn2
  Simulink-PS Converter5/RConn1 -- Revolute Joint4/LConn2
  Simulink-PS Converter6/RConn1 -- Revolute Joint5/LConn2
  Middle1_to4/RConn1 -- Revolute Joint4/LConn1
  Wrist/RConn1 -- Middle1_to6/LConn1

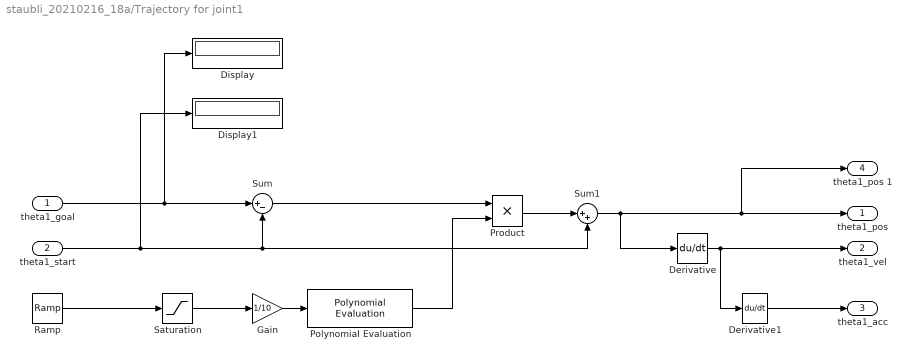
== system staubli_20210216_18a/Trajectory for joint1 ==
  "theta1_goal " : Inport
  "theta1_start " : Inport  Port=2
  Derivative : Derivative
  Derivative1 : Derivative
  Display : Display
  Display1 : Display
  Gain : Gain  Gain=1/10
  Polynomial Evaluation : dsppolyfun/Polynomial Evaluation  useConstCoeffs=on  constCoeffs=[6 -15 10 0 0 0]
      settings: SourceProductBaseCode=DS
  Product : Product
  Ramp : simulink/Sources/Ramp  slope=1  start=0  InitialOutput=0
  Saturation : Saturate  UpperLimit=10  LowerLimit=-10
  Sum : Sum  Inputs=|+-
  Sum1 : Sum  Inputs=|++
  "theta1_pos " : Outport  VectorParamsAs1DForOutWhenUnconnected=off
  "theta1_vel " : Outport  Port=2  VectorParamsAs1DForOutWhenUnconnected=off
  "theta1_acc " : Outport  Port=3  VectorParamsAs1DForOutWhenUnconnected=off
  theta1_pos 1 : Outport  Port=4  VectorParamsAs1DForOutWhenUnconnected=off
  wires:
  "theta1_start "/1 -> Sum1/2, Sum/2, Display1/1
  Sum/1 -> Product/1
  "theta1_goal "/1 -> Display/1, Sum/1
  Sum1/1 -> Derivative/1, theta1_pos 1/1, "theta1_pos "/1
  Derivative/1 -> "theta1_vel "/1, Derivative1/1
  Gain/1 -> Polynomial Evaluation/1
  Product/1 -> Sum1/1
  Polynomial Evaluation/1 -> Product/2
  Derivative1/1 -> "theta1_acc "/1
  Saturation/1 -> Gain/1
  Ramp/1 -> Saturation/1

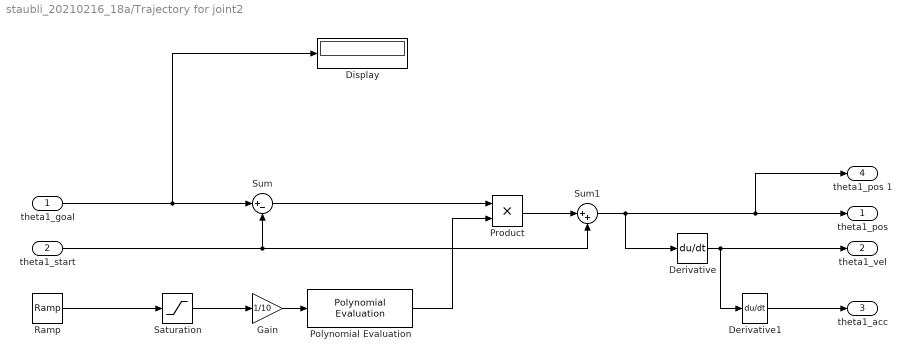
== system staubli_20210216_18a/Trajectory for joint2 ==
  "theta1_goal " : Inport
  "theta1_start " : Inport  Port=2
  Derivative : Derivative
  Derivative1 : Derivative
  Display : Display
  Gain : Gain  Gain=1/10
  Polynomial Evaluation : dsppolyfun/Polynomial Evaluation  useConstCoeffs=on  constCoeffs=[6 -15 10 0 0 0]
      settings: SourceProductBaseCode=DS
  Product : Product
  Ramp : simulink/Sources/Ramp  slope=1  start=0  InitialOutput=0
  Saturation : Saturate  UpperLimit=10  LowerLimit=-10
  Sum : Sum  Inputs=|+-
  Sum1 : Sum  Inputs=|++
  "theta1_pos " : Outport  VectorParamsAs1DForOutWhenUnconnected=off
  "theta1_vel " : Outport  Port=2  VectorParamsAs1DForOutWhenUnconnected=off
  "theta1_acc " : Outport  Port=3  VectorParamsAs1DForOutWhenUnconnected=off
  theta1_pos 1 : Outport  Port=4  VectorParamsAs1DForOutWhenUnconnected=off
  wires:
  "theta1_start "/1 -> Sum1/2, Sum/2
  Sum/1 -> Product/1
  "theta1_goal "/1 -> Display/1, Sum/1
  Sum1/1 -> Derivative/1, theta1_pos 1/1, "theta1_pos "/1
  Derivative/1 -> "theta1_vel "/1, Derivative1/1
  Gain/1 -> Polynomial Evaluation/1
  Product/1 -> Sum1/1
  Polynomial Evaluation/1 -> Product/2
  Derivative1/1 -> "theta1_acc "/1
  Saturation/1 -> Gain/1
  Ramp/1 -> Saturation/1

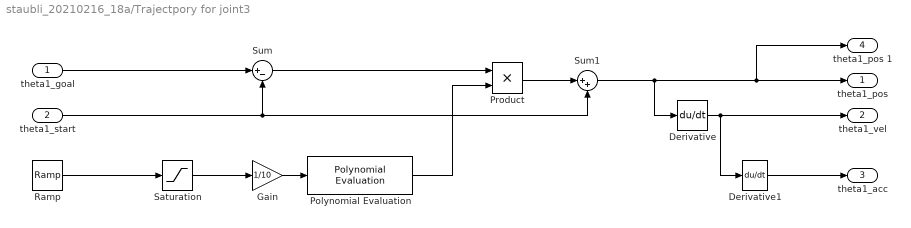
== system staubli_20210216_18a/Trajectpory for joint3 ==
  "theta1_goal " : Inport
  "theta1_start " : Inport  Port=2
  Derivative : Derivative
  Derivative1 : Derivative
  Gain : Gain  Gain=1/10
  Polynomial Evaluation : dsppolyfun/Polynomial Evaluation  useConstCoeffs=on  constCoeffs=[6 -15 10 0 0 0]
      settings: SourceProductBaseCode=DS
  Product : Product
  Ramp : simulink/Sources/Ramp  slope=1  start=0  InitialOutput=0
  Saturation : Saturate  UpperLimit=10  LowerLimit=-10
  Sum : Sum  Inputs=|+-
  Sum1 : Sum  Inputs=|++
  "theta1_pos " : Outport  VectorParamsAs1DForOutWhenUnconnected=off
  "theta1_vel " : Outport  Port=2  VectorParamsAs1DForOutWhenUnconnected=off
  "theta1_acc " : Outport  Port=3  VectorParamsAs1DForOutWhenUnconnected=off
  theta1_pos 1 : Outport  Port=4  VectorParamsAs1DForOutWhenUnconnected=off
  wires:
  Sum/1 -> Product/1
  Derivative/1 -> "theta1_vel "/1, Derivative1/1
  Gain/1 -> Polynomial Evaluation/1
  Product/1 -> Sum1/1
  Polynomial Evaluation/1 -> Product/2
  Derivative1/1 -> "theta1_acc "/1
  Saturation/1 -> Gain/1
  Ramp/1 -> Saturation/1
  "theta1_goal "/1 -> Sum/1
  "theta1_start "/1 -> Sum1/2, Sum/2
  Sum1/1 -> Derivative/1, theta1_pos 1/1, "theta1_pos "/1

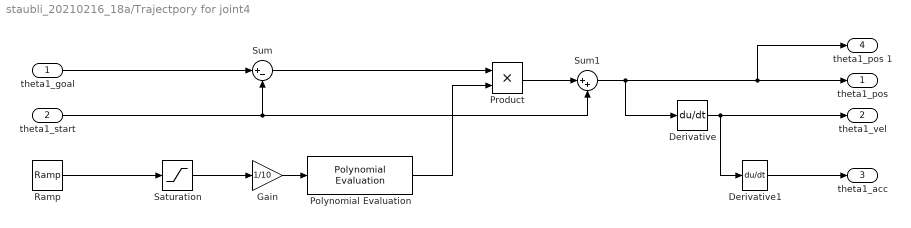
== system staubli_20210216_18a/Trajectpory for joint4 ==
  "theta1_goal " : Inport
  "theta1_start " : Inport  Port=2
  Derivative : Derivative
  Derivative1 : Derivative
  Gain : Gain  Gain=1/10
  Polynomial Evaluation : dsppolyfun/Polynomial Evaluation  useConstCoeffs=on  constCoeffs=[6 -15 10 0 0 0]
      settings: SourceProductBaseCode=DS
  Product : Product
  Ramp : simulink/Sources/Ramp  slope=1  start=0  InitialOutput=0
  Saturation : Saturate  UpperLimit=10  LowerLimit=-10
  Sum : Sum  Inputs=|+-
  Sum1 : Sum  Inputs=|++
  "theta1_pos " : Outport  VectorParamsAs1DForOutWhenUnconnected=off
  "theta1_vel " : Outport  Port=2  VectorParamsAs1DForOutWhenUnconnected=off
  "theta1_acc " : Outport  Port=3  VectorParamsAs1DForOutWhenUnconnected=off
  theta1_pos 1 : Outport  Port=4  VectorParamsAs1DForOutWhenUnconnected=off
  wires:
  "theta1_start "/1 -> Sum1/2, Sum/2
  Sum/1 -> Product/1
  "theta1_goal "/1 -> Sum/1
  Sum1/1 -> Derivative/1, theta1_pos 1/1, "theta1_pos "/1
  Derivative/1 -> "theta1_vel "/1, Derivative1/1
  Gain/1 -> Polynomial Evaluation/1
  Product/1 -> Sum1/1
  Polynomial Evaluation/1 -> Product/2
  Derivative1/1 -> "theta1_acc "/1
  Saturation/1 -> Gain/1
  Ramp/1 -> Saturation/1

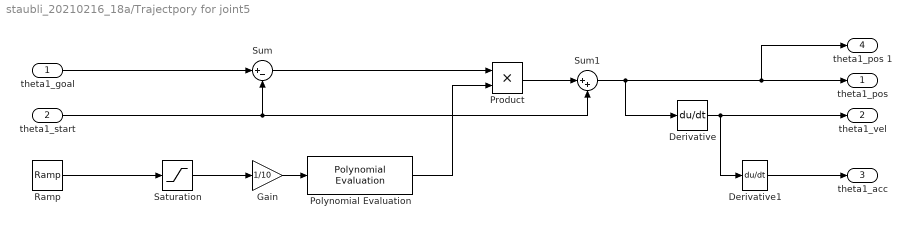
== system staubli_20210216_18a/Trajectpory for joint5 ==
  "theta1_goal " : Inport
  "theta1_start " : Inport  Port=2
  Derivative : Derivative
  Derivative1 : Derivative
  Gain : Gain  Gain=1/10
  Polynomial Evaluation : dsppolyfun/Polynomial Evaluation  useConstCoeffs=on  constCoeffs=[6 -15 10 0 0 0]
      settings: SourceProductBaseCode=DS
  Product : Product
  Ramp : simulink/Sources/Ramp  slope=1  start=0  InitialOutput=0
  Saturation : Saturate  UpperLimit=10  LowerLimit=-10
  Sum : Sum  Inputs=|+-
  Sum1 : Sum  Inputs=|++
  "theta1_pos " : Outport  VectorParamsAs1DForOutWhenUnconnected=off
  "theta1_vel " : Outport  Port=2  VectorParamsAs1DForOutWhenUnconnected=off
  "theta1_acc " : Outport  Port=3  VectorParamsAs1DForOutWhenUnconnected=off
  theta1_pos 1 : Outport  Port=4  VectorParamsAs1DForOutWhenUnconnected=off
  wires:
  "theta1_start "/1 -> Sum1/2, Sum/2
  Sum/1 -> Product/1
  "theta1_goal "/1 -> Sum/1
  Sum1/1 -> Derivative/1, theta1_pos 1/1, "theta1_pos "/1
  Derivative/1 -> "theta1_vel "/1, Derivative1/1
  Gain/1 -> Polynomial Evaluation/1
  Product/1 -> Sum1/1
  Polynomial Evaluation/1 -> Product/2
  Derivative1/1 -> "theta1_acc "/1
  Saturation/1 -> Gain/1
  Ramp/1 -> Saturation/1

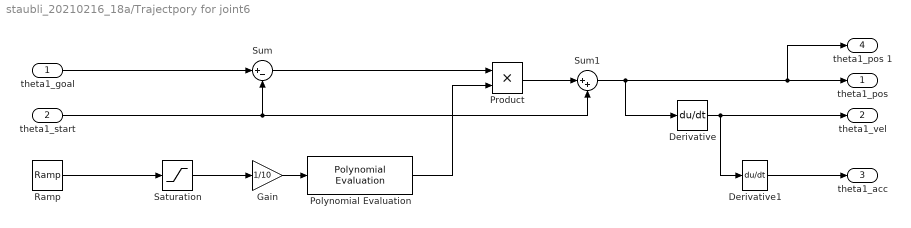
== system staubli_20210216_18a/Trajectpory for joint6 ==
  "theta1_goal " : Inport
  "theta1_start " : Inport  Port=2
  Derivative : Derivative
  Derivative1 : Derivative
  Gain : Gain  Gain=1/10
  Polynomial Evaluation : dsppolyfun/Polynomial Evaluation  useConstCoeffs=on  constCoeffs=[6 -15 10 0 0 0]
      settings: SourceProductBaseCode=DS
  Product : Product
  Ramp : simulink/Sources/Ramp  slope=1  start=0  InitialOutput=0
  Saturation : Saturate  UpperLimit=20  LowerLimit=-20
  Sum : Sum  Inputs=|+-
  Sum1 : Sum  Inputs=|++
  "theta1_pos " : Outport  VectorParamsAs1DForOutWhenUnconnected=off
  "theta1_vel " : Outport  Port=2  VectorParamsAs1DForOutWhenUnconnected=off
  "theta1_acc " : Outport  Port=3  VectorParamsAs1DForOutWhenUnconnected=off
  theta1_pos 1 : Outport  Port=4  VectorParamsAs1DForOutWhenUnconnected=off
  wires:
  "theta1_start "/1 -> Sum1/2, Sum/2
  Sum/1 -> Product/1
  "theta1_goal "/1 -> Sum/1
  Sum1/1 -> Derivative/1, theta1_pos 1/1, "theta1_pos "/1
  Derivative/1 -> "theta1_vel "/1, Derivative1/1
  Gain/1 -> Polynomial Evaluation/1
  Product/1 -> Sum1/1
  Polynomial Evaluation/1 -> Product/2
  Derivative1/1 -> "theta1_acc "/1
  Saturation/1 -> Gain/1
  Ramp/1 -> Saturation/1

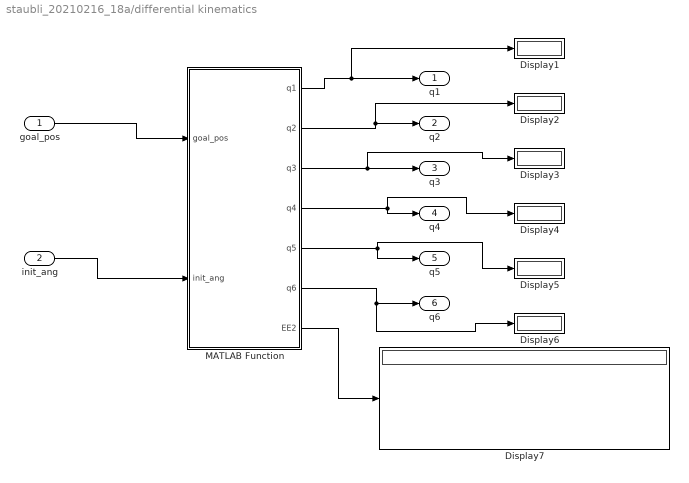
== system staubli_20210216_18a/differential kinematics ==
  goal_pos : Inport
  init_ang : Inport  Port=2
  Display{1..7} (7 alike) : Display
  MATLAB Function : MATLAB Function  TreatAsAtomicUnit=on
  q1 : Outport
  q2 : Outport  Port=2
  q3 : Outport  Port=3
  q4 : Outport  Port=4
  q5 : Outport  Port=5
  q6 : Outport  Port=6
  wires:
  goal_pos/1 -> MATLAB Function/1(goal_pos)
  init_ang/1 -> MATLAB Function/2(init_ang)
  MATLAB Function/2(q2) -> Display2/1, q2/1
  MATLAB Function/3(q3) -> Display3/1, q3/1
  MATLAB Function/4(q4) -> Display4/1, q4/1
  MATLAB Function/5(q5) -> Display5/1, q5/1
  MATLAB Function/6(q6) -> Display6/1, q6/1
  MATLAB Function/1(q1) -> Display1/1, q1/1
  MATLAB Function/7(EE2) -> Display7/1

== matlab function staubli_20210216_18a/differential kinematics/MATLAB Function ==
  data: goal_pos input; q1 output; init_ang input; q2 output; q3 output; q4 output; q5 output; q6 output; EE2 output
function [q1,q2, q3, q4, q5, q6, EE2]= jacobian(goal_pos, init_ang)
theta1=init_ang(1);  d1=0;   a1=50;  alpha1=-90; %parameter link1
theta2=init_ang(2);  d2=0;   a2=425;  alpha2=0; %parameter link2
theta3=init_ang(3);  d3=50;  a3=425;  alpha3=0; %parameter link3
theta4=init_ang(4);  d4=0;   a4=0;  alpha4=90; %parameter link4
theta5=init_ang(5);  d5=100; a5=0;  alpha5=-90; %parameter link5
theta6=init_ang(6);  d6=0; a6=0;  alpha6=90; %parameter link6
offset2 = -90;
offset4 = 90;
% DH paramter 
End_EE = [0 0 0 0;
         0 0 0 0;
         0 0 0 0;
         0 0 0 1];
     
Xc=goal_pos(1);Yc=goal_pos(2);Zc=goal_pos(3);
r=goal_pos(4);p=goal_pos(5);yaw=goal_pos(6);
% init pos and orientation(Euler)

iteration = 0;
b = 0 ;
deltatheta1=0;deltatheta2=0; deltatheta3=0; %theta1,2,3 velocity
deltatheta4=0;deltatheta5=0; deltatheta6=0; %theta1,2,3 velocity
while b == 0
    if theta1 >180
        theta1 = -180 + theta1;
    elseif theta1 <-180
        theta1 = -theta1;
    end
    if theta2 >147.5
        theta2 = -147.5 + theta2;
    elseif theta2 <-130
        theta2 = -theta2;
    end
    if theta3 >145
        theta3 = -145 + theta3;
    elseif theta1 <-145
        theta3 = -theta3;
    end
    if theta4 >270
        theta4 = -270 + theta4;
    elseif theta4 <-270
        theta4 = -theta4;
    end
    if theta5 >140
        theta5 = -140 + theta5;
    elseif theta5 <-115
        theta5 = -theta5;
    end
    if theta6 >270
        theta6 = -270 + theta6;
    elseif theta6 <-270
        theta6 = -theta6;
    end
    result = [theta1 theta2 theta3 theta4 theta5 theta6]
    disp(result)
    theta1=theta1+deltatheta1/2;
    theta2=theta2+deltatheta2/2;
    theta3=theta3+deltatheta3/2;
    theta4=theta4+deltatheta4/2;
    theta5=theta5+deltatheta5/2;
    theta6=theta6+deltatheta6/2;
    if(iteration > 1000)
        % avoid too many calculation
        b=1;
        iteration = 0;
    end
    T01=[cosd(theta1) -cosd(alpha1)*sind(theta1) sind(alpha1)*sind(theta1) a1*cosd(theta1);
        sind(theta1) cosd(alpha1)*cosd(theta1)  -sind(alpha1)*cosd(theta1) a1*sind(theta1);
        0,sind(alpha1),cosd(alpha1),d1;
        0,0,0,1];
    T12=[cosd(theta2+offset2) -cosd(alpha2)*sind(theta2+offset2) sind(alpha2)*sind(theta2+offset2) a2*cosd(theta2+offset2);
        sind(theta2+offset2) cosd(alpha2)*cosd(theta2+offset2)  -sind(alpha2)*cosd(theta2+offset2) a2*sind(theta2+offset2);
        0,sind(alpha2),cosd(alpha2),d2;
        0,0,0,1];
    T23=[cosd(theta3) -cosd(alpha3)*sind(theta3) sind(alpha3)*sind(theta3) a3*cosd(theta3);
        sind(theta3) cosd(alpha3)*cosd(theta3)  -sind(alpha3)*cosd(theta3) a3*sind(theta3);
        0,sind(alpha3),cosd(alpha3),d3;
        0,0,0,1];
    T34=[cosd(theta4+offset4) -cosd(alpha4)*sind(theta4+offset4) sind(alpha4)*sind(theta4+offset4) a4*cosd(theta4+offset4);
         sind(theta4+offset4) cosd(alpha4)*cosd(theta4+offset4)  -sind(alpha4)*cosd(theta4+offset4) a4*sind(theta4+offset4);
         0,sind(alpha4),cosd(alpha4),d4;
         0,0,0,1];
    T45=[cosd(theta5) -cosd(alpha5)*sind(theta5) sind(alpha5)*sind(theta5) a5*cosd(theta5);
         sind(theta5) cosd(alpha5)*cosd(theta5)  -sind(alpha5)*cosd(theta5) a5*sind(theta5);
         0,sind(alpha5),cosd(alpha5),d5;
         0,0,0,1];
    T56=[cosd(theta6) -cosd(alpha6)*sind(theta6) sind(alpha6)*sind(theta6) a6*cosd(theta6);
         sind(theta6) cosd(alpha6)*cosd(theta6)  -sind(alpha6)*cosd(theta6) a6*sind(theta6);
         0,sind(alpha6),cosd(alpha6),d6;
         0,0,0,1];
    T01;
    T02 = T01*T12;
    T03=T01*T12*T23;
    T04=T01*T12*T23*T34;
    T05=T01*T12*T23*T34*T45;
    T06=T01*T12*T23*T34*T45*T56

    P0=[0 0 0];
    P1=transpose(T01(1:3,4));
    P2=transpose(T02(1:3,4));
    P3=transpose(T03(1:3,4));
    P4=transpose(T04(1:3,4));
    P5=transpose(T05(1:3,4));
    P6=transpose(T06(1:3,4));
    %%%%%%%%%%%%%%%%%%%%%%%
    Z0  = [0;0;1];Ori =[0;0;0]; O6=T06(1:3,4);
    Jv1 = cross(Z0,(O6-Ori));
    
    Z1  = T01(1:3,3);Ori_1=T01(1:3,4);
    Jv2 = cross(Z1,(O6-Ori_1));
    
    Z2  = T12(1:3,3);Ori_2=T12(1:3,4);
    Jv3 = cross(Z2,(O6-Ori_2));

    Z3  = T23(1:3,3);Ori_3=T23(1:3,4);
    Jv4 = cross(Z3,(O6-Ori_3));
    
    Z4  = T34(1:3,3);Ori_4=T34(1:3,4);
    Jv5 = cross(Z4,(O6-Ori_4));
    
    Z5  = T45(1:3,3);Ori_5=T45(1:3,4);
    Jv6 = cross(Z5,(O6-Ori_5));
    Jv=[Jv1 Jv2 Jv3 Jv4 Jv5 Jv6];

    Xinit=P6(1,1); 
    Yinit=P6(1,2);
    Zinit = P6(1,3);
    Xend=Xc;Yend=Yc; Zend = Zc;
    Xspeed=(Xend-Xinit);
    Yspeed=(Yend-Yinit);
    Zspeed=(Zend-Zinit);
    thetadot=pinv(Jv)*[Xspeed;Yspeed;Zspeed];
    error_x = Xspeed^2;
    error_z = Yspeed^2;
    error_y = Zspeed^2;
    dis_error=sqrt(error_x+error_y+error_z);
    
    if abs(error_x)<=0.2 && abs(error_y)<=0.2 && abs(error_z)<=0.2
        End_EE = T06;
        b=1;
    end
    theta1dot=thetadot(1,1);
    theta2dot=thetadot(2,1);
    theta3dot=thetadot(3,1);    
    theta4dot=thetadot(4,1);
    theta5dot=thetadot(5,1);
    theta6dot=thetadot(6,1);   
    
    deltatheta1=rad2deg(theta1dot);
    deltatheta2=rad2deg(theta2dot);
    deltatheta3=rad2deg(theta3dot);
    deltatheta4=rad2deg(theta4dot);
    deltatheta5=rad2deg(theta5dot);
    deltatheta6=rad2deg(theta6dot);
    iteration = iteration +1;
end
q1 = theta1;
q2 = theta2;
q3 = theta3;
q4 = theta4;
q5 = theta5;
q6 = theta6;
EE2 = End_EE;
